simulink model "s_cd_ramp"  (R2016b)
(part 2 of 40)

      settings: AttributesFormatString=2 inputs:uf16.0,uf16.0 = 32 bits
      mask TypeOptions io_dir: To Processor | From Processor
      mask Callback io_dir:
      | mask_enables = get_param(gcb, 'MaskEnables');
      | mask_names = get_param(gcb, 'MaskNames');
      | if strcmp(get_param(gcb, 'io_dir'), 'To Processor'),
      |     mask_enables{ismember(mask_names, 'sample_period')} = 'off';
      | else
      |     mask_enables{ismember(mask_names, 'sample_period')} = 'on';
      | end
      | set_param(gcb, 'MaskEnables', mask_enables);
  unpack_and_reorder : Subsystem  mask{n_bits_packet_size=9, n_bits_timestep=9+3, n_bits_fifo_depth=3, n_bits_buffer_depth=4, bram_latency=1}
      mask prompts: n_bits_packet_size "Packet size (2^? 80-bit words after unpacking)"; n_bits_timestep "Packet timestep (2^?)"; n_bits_fifo_depth "FIFO depth (2^? packets)"; n_bits_buffer_depth "Reorder buffer size (2^? packets)"; bram_latency "BRAM latency"
  tag scope: cnt_rst=global
  wires:
  Constant/1 -> port0/1(sim_1)
  port0/1(in_reg) -> Delay16/1
  Constant2/1 -> ip0/1(sim_1)
  ip0/1(in_reg) -> Delay15/1
  Constant3/1 -> forty_gbe/8(rx_overrun_ack)
  Constant4/1 -> forty_gbe/7(rx_ack)
  [gbe_rst] -> forty_gbe/1(rst)
  Delay15/1 -> forty_gbe/4(tx_dest_ip)
  Delay16/1 -> forty_gbe/5(tx_dest_port)
  [sys_rst] -> edge_detect9/1(in)
  bus_expand4/4(lsb_out1) -> [unpack_adc_or1]
  concat0/1 -> unpack_and_reorder/2(din)
  concat1/1 -> unpack_and_reorder/3(eof)
  concat3/1 -> unpack_and_reorder/4(en)
  constant/1 -> unpack_and_reorder/5(transmit)
  unpack_and_reorder/4(timestamp) -> Delay23/1
  unpack_and_reorder/5(recvd) -> bus_expand17/1(bus_in)
  unpack_and_reorder/1(sync) -> Delay12/1
  unpack_and_reorder/2(dout) -> Delay14/1
  unpack_and_reorder/10(discarding) -> Delay44/1
  unpack_and_reorder/11(timestep_error) -> Delay45/1
  sync_gen/2(dout) -> bus_expand6/1(bus_in)
  sync_gen/3(dvalid) -> impulse_gen1/6(en), impulse_gen0/6(en)
  Slice4/1 -> pipeline16/1(d)
  pipeline16/1(q) -> local_time_lsw/1(out_timestamp_lsw)
  Slice16/1 -> Convert6/1
  pipeline47/1(q) -> local_time_msw/1(out_timestamp_msw)
  Convert6/1 -> pipeline47/1(d)
  [time80_48] -> Slice16/1, Slice4/1
  Concat22/1 -> pipeline29/1(d)
  Concat3/1 -> pipeline27/1(d)
  edge_detect9/1(out) -> unpack_and_reorder/1(rst)
  unpack_and_reorder/12(mcnt_relock) -> Delay46/1
  [unpack_recvd0] -> Inverter6/1
  Inverter6/1 -> Logical10/1
  Logical10/1 -> [unpack_missing0]
  [unpack_recvd1] -> Inverter7/1
  unpack_and_reorder/3(dvalid) -> Delay13/1, Logical13/2, Logical10/2
  Inverter7/1 -> Logical13/1
  Logical13/1 -> [unpack_missing1]
  bus_expand17/1(msb_out2) -> [unpack_recvd0]
  bus_expand17/2(lsb_out1) -> [unpack_recvd1]
  Slice12/1 -> [time80]
  impulse_gen0/3(dvalid) -> [valid80]
  impulse_gen0/1(sync_out) -> [sync80]
  impulse_gen0/2(dout) -> [d80_adc0]
  impulse_gen0/4(misco) -> [time80_48], Slice12/1
  [tvg_adc_en] -> impulse_gen0/1(tvg_en)
  impulse_gen1/1(sync_out) -> Terminator6/1
  impulse_gen1/2(dout) -> [d80_adc1]
  impulse_gen1/3(dvalid) -> Terminator8/1
  impulse_gen1/4(misco) -> [dig_flags]
  [tvg_adc_en] -> impulse_gen1/1(tvg_en)
  impulse0/1(in_offset) -> Slice7/1
  impulse0/2(in_amplitude) -> impulse_gen0/3(impulse_amplitude)
  impulse1/1(in_offset) -> Slice8/1
  impulse1/2(in_amplitude) -> impulse_gen1/3(impulse_amplitude)
  sync_gen/1(sync) -> impulse_gen1/4(sync_in), impulse_gen0/4(sync_in)
  bus_expand6/1(msb_out2) -> impulse_gen0/5(din)
  bus_expand6/2(lsb_out1) -> impulse_gen1/5(din)
  sync_gen/5(misco) -> impulse_gen1/7(misci)
  sync_gen/4(time_out) -> impulse_gen0/7(misci)
  Constant31/1 -> Concat9/2
  [unpack_timestamp] -> Concat9/1
  unpack_and_reorder/6(flags) -> Delay24/1
  bus_expand4/1(msb_out4) -> [unpack_ndiode0]
  bus_expand4/2(out3) -> [unpack_adc_or0]
  bus_expand4/3(out2) -> [unpack_ndiode1]
  unpack_and_reorder/7(fifo_of) -> Delay25/1
  Constant8/1 -> Relational3/2
  Relational3/1 -> [unpack_fifo_of]
  Constant34/1 -> Relational4/2
  unpack_and_reorder/8(packet_of) -> Delay48/1, Delay35/1
  Relational4/1 -> [unpack_fifo_pktof]
  Constant35/1 -> Relational5/2
  unpack_and_reorder/9(spead_error) -> Delay47/1, Delay36/1
  Relational5/1 -> [unpack_spead_error]
  Constant36/1 -> Relational6/2
  [unpack_missing0] -> Concat14/1
  [unpack_missing1] -> Concat14/2
  Concat14/1 -> Relational6/1
  Relational6/1 -> [unpack_missing]
  [timestep_error] -> Logical15/1
  [sys_rst] -> Logical15/2
  Logical15/1 -> edge_detect17/1(in)
  edge_detect17/1(out) -> [sys_relock]
  [unpack_fifo_pktof] -> Concat11/5
  [unpack_spead_error] -> Concat11/7
  [unpack_discarding] -> Concat11/4
  [unpack_mcnt_relock] -> Concat11/3
  [unpack_adc_or0] -> Concat11/8
  [unpack_adc_or1] -> Concat11/9
  [unpack_fifo_of] -> Concat11/6
  [unpack_ndiode0] -> Concat11/10
  [unpack_ndiode1] -> Concat11/11
  [unpack_missing] -> Concat11/2
  [timestep_error] -> Concat11/1
  bus_expand18/1(msb_out4) -> [unpack_spead_error0]
  bus_expand18/2(out3) -> [unpack_spead_error1]
  bus_expand18/3(out2) -> [unpack_spead_error2]
  bus_expand18/4(lsb_out1) -> [unpack_spead_error3]
  bus_expand20/1(msb_out4) -> [unpack_fifo_pktof0]
  bus_expand20/2(out3) -> [unpack_fifo_pktof1]
  bus_expand20/3(out2) -> [unpack_fifo_pktof2]
  bus_expand20/4(lsb_out1) -> [unpack_fifo_pktof3]
  phase0/1(in_initial) -> Reinterpret2/1
  delta_delay0/1(in_delta) -> Reinterpret1/1
  phase0/2(in_delta) -> Reinterpret3/1
  Concat9/1 -> sync_gen/1(time_in)
  [sys_relock] -> sync_gen/5(relock)
  Concat11/1 -> sync_gen/4(misci)
  [unpack_en] -> sync_gen/2(en)
  [unpack_d80] -> sync_gen/3(din)
  Delay8/1 -> [unpack_sync]
  Delay9/1 -> [unpack_d80]
  Delay18/1 -> bus_expand4/1(bus_in)
  Delay19/1 -> [unpack_discarding]
  Delay27/1 -> [timestep_error]
  Delay28/1 -> [unpack_mcnt_relock]
  Delay29/1 -> bus_expand18/1(bus_in)
  Delay33/1 -> bus_expand20/1(bus_in)
  Slice7/1 -> impulse_gen0/2(impulse_offset)
  Slice8/1 -> impulse_gen1/2(impulse_offset)
  Delay10/1 -> [unpack_en]
  Delay11/1 -> [unpack_timestamp]
  Reinterpret8/1 -> pipeline56/1(d)
  Reinterpret1/1 -> pipeline55/1(d)
  Reinterpret2/1 -> pipeline54/1(d)
  Reinterpret3/1 -> pipeline53/1(d)
  phase1/1(in_initial) -> Reinterpret5/1
  delta_delay1/1(in_delta) -> Reinterpret4/1
  phase1/2(in_delta) -> Reinterpret6/1
  Reinterpret4/1 -> pipeline51/1(d)
  Reinterpret5/1 -> pipeline50/1(d)
  Reinterpret6/1 -> pipeline49/1(d)
  Reinterpret7/1 -> pipeline52/1(d)
  delay0/1(in_initial) -> Reinterpret8/1
  delay1/1(in_initial) -> Reinterpret7/1
  Delay12/1 -> Delay8/1
  Delay14/1 -> Delay9/1
  Delay13/1 -> Delay10/1
  Delay23/1 -> Delay11/1
  Delay24/1 -> Delay18/1
  Delay25/1 -> Relational3/1
  Delay36/1 -> Relational5/1
  Delay35/1 -> Relational4/1
  Delay46/1 -> Delay28/1
  Delay44/1 -> Delay19/1
  Delay45/1 -> Delay27/1
  Delay47/1 -> Delay29/1
  Delay48/1 -> Delay33/1
  trig_time_msw/1(in_msw) -> pipeline28/1(d)
  trig_time_lsw/1(in_lsw) -> pipeline44/1(d)
  Concat13/1 -> Relational10/1
  pipeline28/1(q) -> Concat13/1
  pipeline44/1(q) -> Concat13/2
  [valid80] -> Counter/2
  [sync80] -> Counter/1
  Constant12/1 -> Relational7/2
  Counter/1 -> Relational7/1
  Relational10/1 -> Mux/2
  Relational7/1 -> Mux/3
  [valid80] -> Delay49/1
  Logical12/1 -> Logical14/1
  Logical14/1 -> [adc_snap_trig]
  [adc_snap_arm] -> Logical14/2
  [time80_48] -> Relational10/2
  Delay49/1 -> Logical12/2
  Mux/1 -> Logical12/1
  [adc_snap_trig_source] -> Mux/1
  Constant10/1 -> iptx_base/1(sim_1)
  Constant9/1 -> tx_metadata/1(sim_1)
  Constant13/1 -> tx_metadata/2(sim_2)
  iptx_base/1(in_reg) -> pipeline105/1(d)
  pipeline105/1(q) -> [tx_ip_base]
  tx_metadata/1(in_porttx) -> pipeline106/1(d)
  tx_metadata/2(in_board_id) -> pipeline107/1(d)
  pipeline106/1(q) -> [tx_port]
  pipeline107/1(q) -> [tx_board_id]
  edge_detect4/1(out) -> pipeline5/1(d)
  control1/6(in_cnt_rst) -> edge_detect1/1(in)
  edge_detect1/1(out) -> pipeline14/1(d)
  control1/3(in_gbe_rst) -> pipeline6/1(d)
  control1/1(in_sys_rst) -> pipeline3/1(d)
  pipeline3/1(q) -> [sys_rst]
  pipeline5/1(q) -> [clr_status]
  pipeline6/1(q) -> [gbe_rst]
  pipeline7/1(q) -> [gbe_txen]
  pipeline13/1(q) -> [tvg_adc_en]
  pipeline14/1(q) -> [cnt_rst]
  control1/5(in_tvg_adc) -> pipeline13/1(d)
  edge_detect2/1(out) -> pipeline38/1(d)
  pipeline38/1(q) -> [gbe_cnt_rst]
  control1/7(in_gbe_cnt_rst) -> edge_detect2/1(in)
  control1/4(in_gbe_txen) -> pipeline7/1(d)
  control1/2(in_status_clr) -> edge_detect4/1(in)
  pipeline43/1(q) -> [adc_snap_arm]
  control1/8(in_adc_snap_arm) -> pipeline43/1(d)
  control1/9(in_adc_snap_trig_select) -> pipeline39/1(d)
  pipeline39/1(q) -> [adc_snap_trig_source]
  Concat4/1 -> concat0/1
  Constant14/1 -> din_reg_0/1(sim_1)
  din_reg_0/1(in_reg) -> pipeline1/1(d)
  Constant15/1 -> din_reg_1/1(sim_1)
  din_reg_1/1(in_reg) -> pipeline2/1(d)
  pipeline1/1(q) -> Concat4/1
  pipeline2/1(q) -> Concat4/2
  Constant16/1 -> din_reg_2/1(sim_1)
  din_reg_2/1(in_reg) -> pipeline4/1(d)
  Constant17/1 -> din_reg_3/1(sim_1)
  din_reg_3/1(in_reg) -> pipeline8/1(d)
  pipeline4/1(q) -> Concat6/1
  pipeline8/1(q) -> Concat6/2
  Concat6/1 -> concat0/2
  Constant18/1 -> din_reg_4/1(sim_1)
  din_reg_4/1(in_reg) -> pipeline9/1(d)
  Constant19/1 -> din_reg_5/1(sim_1)
  din_reg_5/1(in_reg) -> pipeline10/1(d)
  pipeline9/1(q) -> Concat7/1
  pipeline10/1(q) -> Concat7/2
  Concat7/1 -> concat0/3
  Constant20/1 -> din_reg_6/1(sim_1)
  din_reg_6/1(in_reg) -> pipeline12/1(d)
  Constant21/1 -> din_reg_7/1(sim_1)
  din_reg_7/1(in_reg) -> pipeline11/1(d)
  pipeline12/1(q) -> Concat8/1
  pipeline11/1(q) -> Concat8/2
  Concat8/1 -> concat0/4
  Constant22/1 -> eof_reg/1(sim_1)
  eof_reg/1(in_reg) -> pipeline15/1(d)
  pipeline15/1(q) -> bus_expand9/1(bus_in)
  bus_expand9/1(msb_out4) -> concat1/1
  bus_expand9/2(out3) -> concat1/2
  bus_expand9/3(out2) -> concat1/3
  bus_expand9/4(lsb_out1) -> concat1/4
  Constant23/1 -> en_reg/1(sim_1)
  en_reg/1(in_reg) -> pipeline17/1(d)
  pipeline17/1(q) -> bus_expand10/1(bus_in)
  bus_expand10/1(msb_out4) -> concat3/1
  bus_expand10/2(out3) -> concat3/2
  bus_expand10/3(out2) -> concat3/3
  bus_expand10/4(lsb_out1) -> concat3/4
  Delay54/1 -> edge_detect3/1
  Counter5/1 -> Gateway Out3/1, Relational1/1
  Constant32/1 -> Relational1/2
  Delay55/1 -> Delay56/1
  Delay56/1 -> Delay1/1
  Relational1/1 -> [sync80_local], Gateway Out1/1
  edge_detect3/1 -> Gateway Out2/1, Counter5/1
  [ld_val0] -> pipeline23/1(d)
  [clr_status] -> pipeline22/1(d)
  tl_cd0/6(time) -> Terminator16/1
  tl_cd0/3(sync_out) -> pipeline41/1(d)
  tl_cd0/4(dout) -> pipeline42/1(d)
  tl_cd0/5(dvalid) -> pipeline45/1(d)
  tl_cd0/1(value) -> pipeline46/1(d)
  tl_cd0/2(enable) -> pipeline48/1(d)
  cd_compensation0/5(parity_error) -> pipeline86/1(d)
  cd_compensation0/4(hmc_error) -> pipeline85/1(d)
  Constant6/1 -> Concat15/2
  Concat15/1 -> pipeline21/1(d)
  [time80] -> Concat15/1
  Counter2/1 -> pipeline31/1(d)
  Counter4/1 -> pipeline32/1(d)
  Counter9/1 -> pipeline33/1(d)
  Counter10/1 -> pipeline34/1(d)
  Counter11/1 -> pipeline35/1(d)
  Counter12/1 -> pipeline36/1(d)
  Counter14/1 -> pipeline40/1(d)
  Counter13/1 -> pipeline37/1(d)
  Constant7/1 -> delay0/1(sim_1)
  cd_compensation0/2(dout) -> pipeline83/1(d)
  cd_compensation0/1(sync_out) -> pipeline82/1(d)
  cd_compensation0/3(dvalid) -> pipeline84/1(d)
  hmc_error/1(sim_out) -> Terminator9/1
  Convert7/1 -> hmc_error/1(out_reg)
  hmc_parity/1(sim_out) -> Terminator11/1
  Convert8/1 -> hmc_parity/1(out_reg)
  [hmc_error] -> Convert7/1
  [hmc_parity] -> Convert8/1
  Constant11/1 -> dvalid/1(sim_1)
  [valid80] -> Logical/1
  dvalid/1(in_reg) -> pipeline20/1(d)
  pipeline20/1(q) -> Logical/2
  [valid80_local] -> pipeline58/1(d), pipeline59/1(d), pipeline60/1(d), pipeline61/1(d), pipeline62/1(d), pipeline63/1(d), pipeline64/1(d), pipeline65/1(d), pipeline66/1(d)
  Logical/1 -> Delay54/1, Delay55/1
  [cd_in] -> pipeline25/1(d)
  bus_create1/1(bus_out) -> [cd_in]
  pipeline22/1(q) -> tl_cd0/1(rst)
  pipeline21/1(q) -> tl_cd0/2(current_time)
  pipeline23/1(q) -> tl_cd0/3(load_value)
  pipeline24/1(q) -> Gateway Out14/1, tl_cd0/4(sync_in)
  pipeline25/1(q) -> Gateway Out10/1, tl_cd0/5(din)
  pipeline26/1(q) -> Gateway Out11/1, tl_cd0/6(en)
  [sync80] -> Terminator7/1
  [sync80_local] -> pipeline24/1(d)
  [valid80] -> Terminator10/1
  [valid80_cd] -> Gateway Out8/1, pipeline26/1(d)
  Gateway Out10/1 -> To Workspace6/1
  Gateway Out11/1 -> To Workspace7/1
  Gateway Out14/1 -> To Workspace8/1
  Gateway Out15/1 -> To Workspace9/1
  pipeline31/1(q) -> Gateway Out7/1, bus_create1/1(in1)
  pipeline32/1(q) -> bus_create1/2(in2)
  pipeline33/1(q) -> bus_create1/3(in3)
  pipeline34/1(q) -> bus_create1/4(in4)
  pipeline35/1(q) -> bus_create1/5(in5)
  pipeline36/1(q) -> bus_create1/6(in6)
  pipeline37/1(q) -> bus_create1/7(in7)
  pipeline40/1(q) -> bus_create1/8(in8)
  pipeline41/1(q) -> cd_compensation0/1(sync_in)
  pipeline42/1(q) -> cd_compensation0/2(din)
  pipeline45/1(q) -> cd_compensation0/3(en)
  pipeline48/1(q) -> cd_compensation0/5(load_val)
  pipeline46/1(q) -> cd_compensation0/4(delay_val)
  Gateway Out7/1 -> To Workspace3/1
  Gateway Out8/1 -> To Workspace4/1
  Delay2/1 -> pipeline30/1(d)
  pipeline30/1(q) -> [valid80_cd]
  Constant24/1 -> forty_gbe/2(tx_data)
  Constant25/1 -> forty_gbe/3(tx_valid)
  Constant26/1 -> forty_gbe/6(tx_end_of_frame)
  pipeline27/1(q) -> [ld_val1]
  pipeline29/1(q) -> [ld_val0]
  pipeline49/1(q) -> Concat3/4
  pipeline50/1(q) -> Concat3/3
  pipeline51/1(q) -> Concat3/2
  pipeline52/1(q) -> Concat3/1
  pipeline53/1(q) -> Concat22/4
  pipeline54/1(q) -> Concat22/3
  pipeline55/1(q) -> Concat22/2
  pipeline56/1(q) -> Concat22/1
  bus_expand1/8(lsb_out1) -> pipeline176/1(d)  "hmc_out16"
  pipeline222/1(q) -> bus_expand1/1(bus_in)
  [cd_in] -> pipeline222/1(d)
  pipeline176/1(q) -> cd_in/8(in_d07)
  pipeline175/1(q) -> cd_in/7(in_d06)
  pipeline172/1(q) -> cd_in/6(in_d05)
  pipeline171/1(q) -> cd_in/5(in_d04)
  pipeline170/1(q) -> cd_in/4(in_d03)
  pipeline169/1(q) -> cd_in/3(in_d02)
  pipeline168/1(q) -> cd_in/2(in_d01)
  bus_expand1/7(out2) -> pipeline175/1(d)
  bus_expand1/5(out4) -> pipeline171/1(d)
  bus_expand1/4(out5) -> pipeline170/1(d)
  bus_expand1/6(out3) -> pipeline172/1(d)
  bus_expand1/3(out6) -> pipeline169/1(d)
  bus_expand1/2(out7) -> pipeline168/1(d)
  sync_en_cd_in/1(in_reg) -> pipeline224/1(d)
  pipeline223/1(q) -> pipeline178/1(d), pipeline227/1(d)
  [sync_trig] -> Logical29/2
  edge_detect16/1(out) -> Logical29/1
  Logical29/1 -> pipeline177/1(d), pipeline226/1(d)
  Logical30/1 -> edge_detect16/1(in)
  pipeline224/1(q) -> Logical30/2
  pipeline225/1(q) -> Logical30/1
  [sync80_local] -> pipeline225/1(d)
  [valid80_cd] -> pipeline223/1(d)
  pipeline226/1(q) -> cd_in/12(trig)
  pipeline227/1(q) -> cd_in/11(we)
  pipeline178/1(q) -> cd_in/9(in_dvalid)
  pipeline177/1(q) -> cd_in/10(in_sync)
  bus_expand1/1(msb_out8) -> pipeline57/1(d)
  pipeline57/1(q) -> cd_in/1(in_d00)
  pipeline58/1(q) -> Counter2/1
  pipeline59/1(q) -> Counter4/1
  pipeline60/1(q) -> Counter9/1
  pipeline61/1(q) -> Counter10/1
  pipeline62/1(q) -> Counter11/1
  pipeline63/1(q) -> Counter12/1
  pipeline64/1(q) -> Counter13/1
  pipeline65/1(q) -> Counter14/1
  pipeline66/1(q) -> Delay2/1
  bus_expand2/1(msb_out8) -> pipeline167/1(d)  "hmc_out9"
  bus_expand2/8(lsb_out1) -> pipeline73/1(d)  "hmc_out16"
  pipeline76/1(q) -> bus_expand2/1(bus_in)
  [cd_out] -> pipeline76/1(d)
  pipeline73/1(q) -> cd_out/8(in_d07)
  pipeline72/1(q) -> cd_out/7(in_d06)
  pipeline71/1(q) -> cd_out/6(in_d05)
  pipeline70/1(q) -> cd_out/5(in_d04)
  pipeline69/1(q) -> cd_out/4(in_d03)
  pipeline68/1(q) -> cd_out/3(in_d02)
  pipeline67/1(q) -> cd_out/2(in_d01)
  pipeline167/1(q) -> cd_out/1(in_d00)
  bus_expand2/7(out2) -> pipeline72/1(d)
  bus_expand2/5(out4) -> pipeline70/1(d)
  bus_expand2/4(out5) -> pipeline69/1(d)
  bus_expand2/6(out3) -> pipeline71/1(d)
  bus_expand2/3(out6) -> pipeline68/1(d)
  bus_expand2/2(out7) -> pipeline67/1(d)
  sync_en_cd_out/1(in_reg) -> pipeline78/1(d)
  pipeline77/1(q) -> pipeline75/1(d), pipeline81/1(d)
  [sync_trig] -> Logical1/2
  edge_detect5/1(out) -> Logical1/1
  Logical1/1 -> pipeline74/1(d), pipeline80/1(d)
  Logical2/1 -> edge_detect5/1(in)
  pipeline78/1(q) -> Logical2/2
  pipeline79/1(q) -> Logical2/1
  [cd_sync] -> pipeline79/1(d)
  [cd_dvalid] -> pipeline77/1(d)
  pipeline80/1(q) -> cd_out/12(trig)
  pipeline81/1(q) -> cd_out/11(we)
  pipeline75/1(q) -> cd_out/9(in_dvalid)
  pipeline74/1(q) -> cd_out/10(in_sync)
  pipeline82/1(q) -> [cd_sync]
  pipeline83/1(q) -> [cd_out]
  pipeline84/1(q) -> [cd_dvalid]
  pipeline85/1(q) -> [hmc_error]
  pipeline86/1(q) -> [hmc_parity]
  Gateway Out1/1 -> To Workspace1/1
  Gateway Out3/1 -> To Workspace5/1
  Gateway Out2/1 -> To Workspace2/1
  Delay1/1 -> Delay3/1
  Delay3/1 -> [valid80_local], Gateway Out15/1
